simulink library "INT_FanCtl_Spd"  (R2016b)
settings: Solver=VariableStepAuto  StartTime=0.0  StopTime=10.0  RelTol=1e-3
settings Model: Creator=liutao  LastModifiedBy=liutao

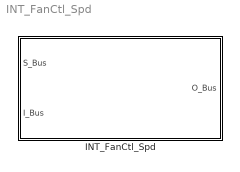
== system INT_FanCtl_Spd ==
  INT_FanCtl_Spd : Subsystem

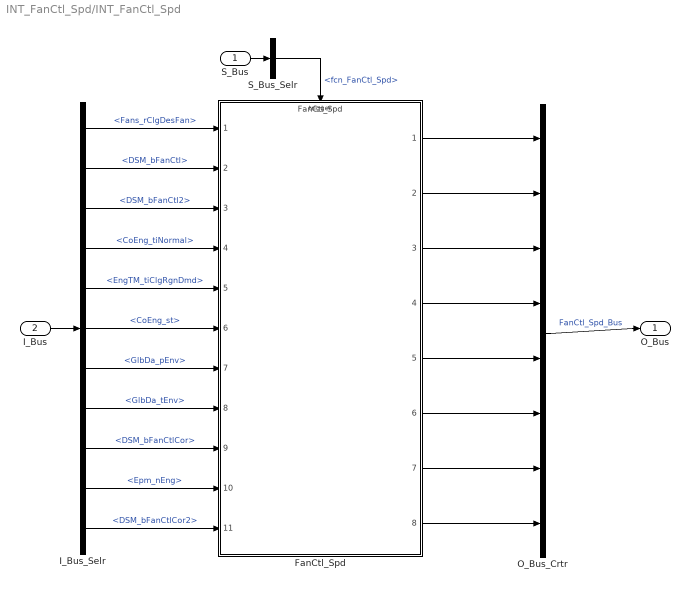
== system INT_FanCtl_Spd/INT_FanCtl_Spd ==
  S_Bus : Inport
  I_Bus : Inport  Port=2
  FanCtl_Spd : ModelReference  ModelNameDialog=FanCtl_Spd  SimulationMode=Normal  ModelReferenceVersion=1.198  TriggerPortName=function  TriggerPortTriggerType=function-call  TriggerPortStatesWhenEnabling=held
  I_Bus_Selr : BusSelector  OutputSignals=Fans_rClgDesFan,DSM_bFanCtl,DSM_bFanCtl2,CoEng_tiNormal,EngTM_tiClgRgnDmd,CoEng_st,GlbDa_pEnv,GlbDa_tEnv,DSM_bFanCtlCor,Epm_nEng,DSM_bFanCtlCor2
  O_Bus_Crtr : BusCreator  Inputs=8
  S_Bus_Selr : BusSelector  OutputSignals=fcn_FanCtl_Spd
  O_Bus : Outport
  wires:
  S_Bus_Selr/1 -> FanCtl_Spd/Trigger  "<fcn_FanCtl_Spd>"
  S_Bus/1 -> S_Bus_Selr/1
  I_Bus/1 -> I_Bus_Selr/1
  I_Bus_Selr/1 -> FanCtl_Spd/1  "<Fans_rClgDesFan>"
  I_Bus_Selr/2 -> FanCtl_Spd/2  "<DSM_bFanCtl>"
  I_Bus_Selr/3 -> FanCtl_Spd/3  "<DSM_bFanCtl2>"
  I_Bus_Selr/4 -> FanCtl_Spd/4  "<CoEng_tiNormal>"
  I_Bus_Selr/5 -> FanCtl_Spd/5  "<EngTM_tiClgRgnDmd>"
  I_Bus_Selr/6 -> FanCtl_Spd/6  "<CoEng_st>"
  I_Bus_Selr/7 -> FanCtl_Spd/7  "<GlbDa_pEnv>"
  I_Bus_Selr/8 -> FanCtl_Spd/8  "<GlbDa_tEnv>"
  I_Bus_Selr/9 -> FanCtl_Spd/9  "<DSM_bFanCtlCor>"
  I_Bus_Selr/10 -> FanCtl_Spd/10  "<Epm_nEng>"
  I_Bus_Selr/11 -> FanCtl_Spd/11  "<DSM_bFanCtlCor2>"
  O_Bus_Crtr/1 -> O_Bus/1  "FanCtl_Spd_Bus"
  FanCtl_Spd/1 -> O_Bus_Crtr/1
  FanCtl_Spd/2 -> O_Bus_Crtr/2
  FanCtl_Spd/3 -> O_Bus_Crtr/3
  FanCtl_Spd/4 -> O_Bus_Crtr/4
  FanCtl_Spd/5 -> O_Bus_Crtr/5
  FanCtl_Spd/6 -> O_Bus_Crtr/6
  FanCtl_Spd/7 -> O_Bus_Crtr/7
  FanCtl_Spd/8 -> O_Bus_Crtr/8
